simulink model "psbpiline"  (Simulink 6.0)
settings: Solver=ode15s  SolverMode=SingleTasking  StartTime=0.0  StopTime=0.05  RelTol=1e-3  AbsTol=1e-6
libraries: powerlib2 x10
settings Model: Creator=patrice  LastModifiedBy=batserve  ExtModeTrigMode=oneshot  ExtModeArmWhenConnect=off  ExtModeAutoUpdateStatusClock=off
settings DataIOCC: LimitDataPoints=off  SignalLoggingName=sigsOut
settings OptimizationCC: BooleanDataType=off
settings DebuggingCC: SolverPrmCheckMsg=none
settings HardwareCC: TargetUnknown=on
settings RTWCC: TemplateMakefile=grt_unix.tmf

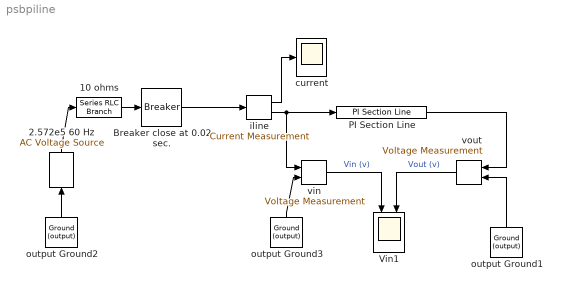
== system psbpiline ==
  10 ohms : powerlib2/Elements/Series RLC Branch  Tag=PoWeRsYsTeMbLoCk  a=10  b=0  c=inf  mesure=None  PSBOutputType=1
  "2.572e5 60 Hz " : powerlib2/Electrical Sources/AC Voltage Source  Tag=PoWeRsYsTeMbLoCk  Orientation=up  A=(315e3*sqrt(2))/sqrt(30)  P=0  F=60  stime=0  mesure=None  PSBOutputType=1
  Breaker close at 0.02 sec. : powerlib2/Elements/Breaker  Tag=PoWeRsYsTeMbLoCk  a=1e-1  c=0  rs=inf  cs=0  times=[ .02 ]  Ts=0  comext=off  mesure=None  PSBOutputType=1
  PI Section Line : powerlib2/Elements/PI Section Line  Tag=PoWeRsYsTeMbLoCk  f=60  a=0.2568  b=2e-03  c=8.6e-09  d=100  e=1  mesure=None  PSBOutputType=1
  Vin1 : Scope  NumInputPorts=2
      settings: Orientation=down  TickLabels=on  TimeRange=0.05  YMin=-100000~-5  YMax=100000~5  DataFormat=Array
  current : Scope
      settings: TickLabels=on  TimeRange=0.05  YMin=-100  YMax=100  DataFormat=Array  MaxDataPoints=5000000
  iline : powerlib2/Measurements/Current Measurement  Tag=PoWeRsYsTeMmEaSuReMeNt  PhasorSimulation=off  OutputType=Magnitude  PSBOutputType=01  PSBequivalent=0
  output Ground1 : powerlib2/Connectors/Ground (output)  Tag=PoWeRsYsTeMbLoCk  Orientation=up  PSBOutputType=1
  output Ground2 : powerlib2/Connectors/Ground (output)  Tag=PoWeRsYsTeMbLoCk  Orientation=up  PSBOutputType=1
  output Ground3 : powerlib2/Connectors/Ground (output)  Tag=PoWeRsYsTeMbLoCk  Orientation=up  PSBOutputType=1
  vin : powerlib2/Measurements/Voltage Measurement  Tag=PoWeRsYsTeMmEaSuReMeNt  PhasorSimulation=off  OutputType=Magnitude  PSBOutputType=0  PSBequivalent=0
  vout : powerlib2/Measurements/Voltage Measurement  Tag=PoWeRsYsTeMmEaSuReMeNt  Orientation=left  PhasorSimulation=off  OutputType=Magnitude  PSBOutputType=0  PSBequivalent=0
  wires:
  "2.572e5 60 Hz "/1 -> 10 ohms/1
  10 ohms/1 -> Breaker close at 0.02 sec./1
  output Ground2/1 -> "2.572e5 60 Hz "/1
  PI Section Line/1 -> vout/1
  iline/1 -> current/1
  output Ground1/1 -> vout/2
  Breaker close at 0.02 sec./1 -> iline/1
  output Ground3/1 -> vin/2
  iline/2 -> PI Section Line/1, vin/1
  vin/1 -> Vin1/1  "Vin (v)"
  vout/1 -> Vin1/2  "Vout (v)"
